simulink model "conv_coding"  (R2016a)
settings: Solver=VariableStepAuto  StartTime=0.0  StopTime=inf  RelTol=1e-3
undefined symbols (not defined in the file or in its folder): randseed
libraries: commcnvcod2 x2, commrandsrc3 x1, commchan3 x1, commsink2 x1
settings Model: Creator=dw  LastModifiedBy=dw

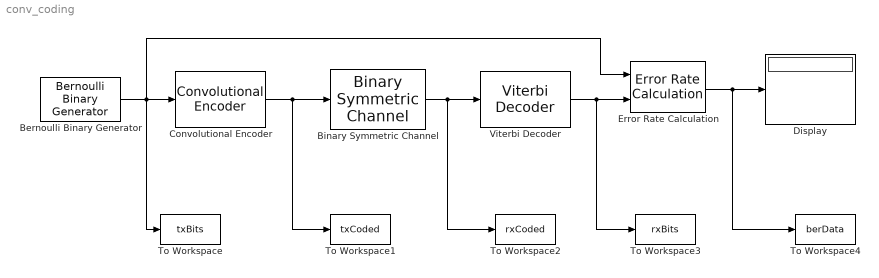
== system conv_coding ==
  Bernoulli Binary Generator : commrandsrc3/Bernoulli Binary Generator  ProbabilityOfZero=0.5  SeedSource=Parameter  Seed=randseed  SampleTime=1  SamplesPerFrame=2  OutputDataType=double  SimulateUsing=Interpreted execution
  Binary Symmetric Channel : commchan3/Binary Symmetric Channel  P=0.02  s=randseed  E=off  outDtype=double
  Convolutional Encoder : commcnvcod2/Convolutional Encoder  trellis=poly2trellis([5 4], [27 33 0; 0 5 13])  opMode=Continuous  DelayedResetAction=off  hasIniStPort=off  hasFinStPort=off  usePuncVector=off  punctureVector=[1; 1; 0; 1; 0; 1]  reset=Unused parameter value
  Display : Display
  Error Rate Calculation : commsink2/Error Rate Calculation  N=68  st_delay=0  cp_mode=Entire frame  subframe=[]  PMode=Port  WsName=ErrorVec  RsMode2=off  stop=on  numErr=100  maxBits=1e6
  To Workspace : ToWorkspace  VariableName=txBits  SaveFormat=Timeseries  SampleTime=-1
  To Workspace1 : ToWorkspace  VariableName=txCoded  SaveFormat=Timeseries  SampleTime=-1
  To Workspace2 : ToWorkspace  VariableName=rxCoded  SaveFormat=Timeseries  SampleTime=-1
  To Workspace3 : ToWorkspace  VariableName=rxBits  SaveFormat=Timeseries  SampleTime=-1
  To Workspace4 : ToWorkspace  VariableName=berData  SaveFormat=Timeseries  SampleTime=-1
  Viterbi Decoder : commcnvcod2/Viterbi Decoder  trellis=poly2trellis([5 4], [27 33 0; 0 5 13])  isPunctured=off  punctureVector=[1; 1; 0; 1; 0; 1]  erasures=off  dectype=Hard decision  nsdecb=4  runSigValErrCheck=off  tbdepth=34  opmode=Continuous  reset=off  delayedResetAction=off  smWordLength=16  outDataType=Inherit via internal rule
  wires:
  Convolutional Encoder/1 -> To Workspace1/1, Binary Symmetric Channel/1
  Bernoulli Binary Generator/1 -> To Workspace/1, Error Rate Calculation/1, Convolutional Encoder/1
  Binary Symmetric Channel/1 -> To Workspace2/1, Viterbi Decoder/1
  Viterbi Decoder/1 -> To Workspace3/1, Error Rate Calculation/2
  Error Rate Calculation/1 -> To Workspace4/1, Display/1
